simulink model "WiberSystem"  (R2023b)
settings: Solver=VariableStepAuto  StartTime=0.0  StopTime=10.0  RelTol=1e-3
settings Model: Creator=MOHAMED  LastModifiedBy=MOHAMED

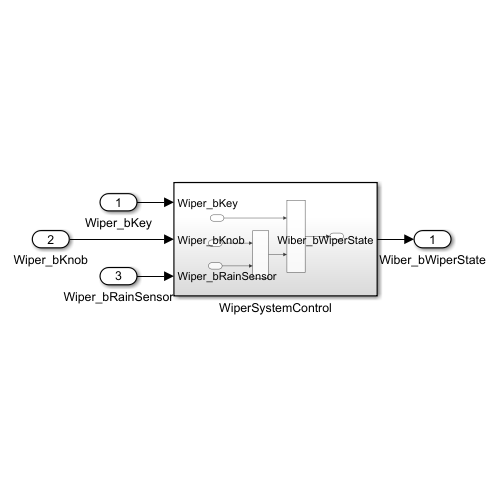
[thumbnail: Simulink's stored preview of the top-level diagram]
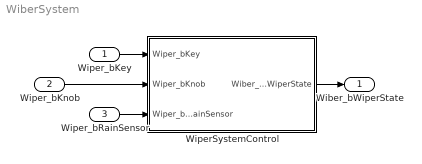
== system WiberSystem ==
  Wiper_bKey : Inport
  Wiper_bKnob : Inport  Port=2
  Wiper_bRainSensor : Inport  Port=3
  WiperSystemControl : Subsystem
  Wiber_bWiperState : Outport
  wires:
  WiperSystemControl/1(Wiber_bWiperState) -> Wiber_bWiperState/1
  Wiper_bRainSensor/1 -> WiperSystemControl/3(Wiper_bRainSensor)
  Wiper_bKnob/1 -> WiperSystemControl/2(Wiper_bKnob)
  Wiper_bKey/1 -> WiperSystemControl/1(Wiper_bKey)

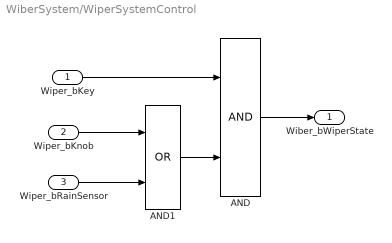
== system WiberSystem/WiperSystemControl ==
  Wiper_bKey : Inport
  Wiper_bKnob : Inport  Port=2
  Wiper_bRainSensor : Inport  Port=3
  AND : Logic  AllPortsSameDT=off  OutDataTypeStr=boolean
  AND1 : Logic  Operator=OR  AllPortsSameDT=off  OutDataTypeStr=boolean
  Wiber_bWiperState : Outport
  wires:
  Wiper_bKnob/1 -> AND1/1
  Wiper_bRainSensor/1 -> AND1/2
  Wiper_bKey/1 -> AND/1
  AND1/1 -> AND/2
  AND/1 -> Wiber_bWiperState/1
